simulink model "System_Analysis_for_no_P_and_PI_Controllers"  (R2023a)
settings: Solver=FixedStepDiscrete  StartTime=0.0  StopTime=100  FixedStep=0.001  RelTol=1e-3  EnableMultiTasking=on
undefined symbols (not defined in the file or in its folder): DiscIntNeverNeededParam
libraries: arduinolib x6
settings Model: ExtModeTrigDuration=2  Creator=Mohamed Ezzelrgal  LastModifiedBy=Mohamed Ezzelrgal
settings OptimizationCC: EnhancedBackFolding=on  PassReuseOutputArgsAs=Individual arguments  ZeroExternalMemoryAtStartup=off  ZeroInternalMemoryAtStartup=off  MaxStackSize=64  OptimizeBlockOrder=speed  DifferentSizesBufferReuse=on  OptimizationCustomize=off  EfficientTunableParamExpr=on
settings DebuggingCC: ParameterTunabilityLossMsg=error
settings HardwareCC: ProdBitPerInt=16  ProdBitPerPointer=16  ProdBitPerSizeT=16  ProdBitPerPtrDiffT=16  ProdLargestAtomicFloat=None  ProdWordSize=8  ProdHWDeviceType=Atmel->AVR
settings SFSimCC: MATLABDynamicMemAlloc=off
settings RTWCC: Description=Embedded Coder  SystemTargetFile=ert.tlc  HardwareBoard=Arduino Uno  TemplateMakefile=ert_default_tmf  Toolchain=Arduino AVR  BuildConfiguration=Faster Runs
settings CodeAppCC: ForceParamTrailComments=on  IgnoreCustomStorageClasses=off  OperatorAnnotations=on  SimulinkDataObjDesc=on  SFDataObjDesc=on  InsertBlockDesc=on
settings ERTTargetCC: SupportContinuousTime=on  SupportVariableSizeSignals=on  ExtModeTransport=3  ExtModeStaticAlloc=on  ExtModeAutomaticAllocSize=off  ExtModeStaticAllocSize=250  ExtModeMexFile=ext_xcp  ExtModeIntrfLevel=Level2 - Open

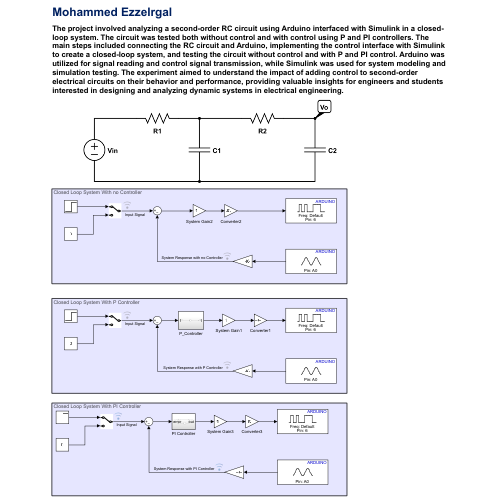
[thumbnail: Simulink's stored preview of the top-level diagram]
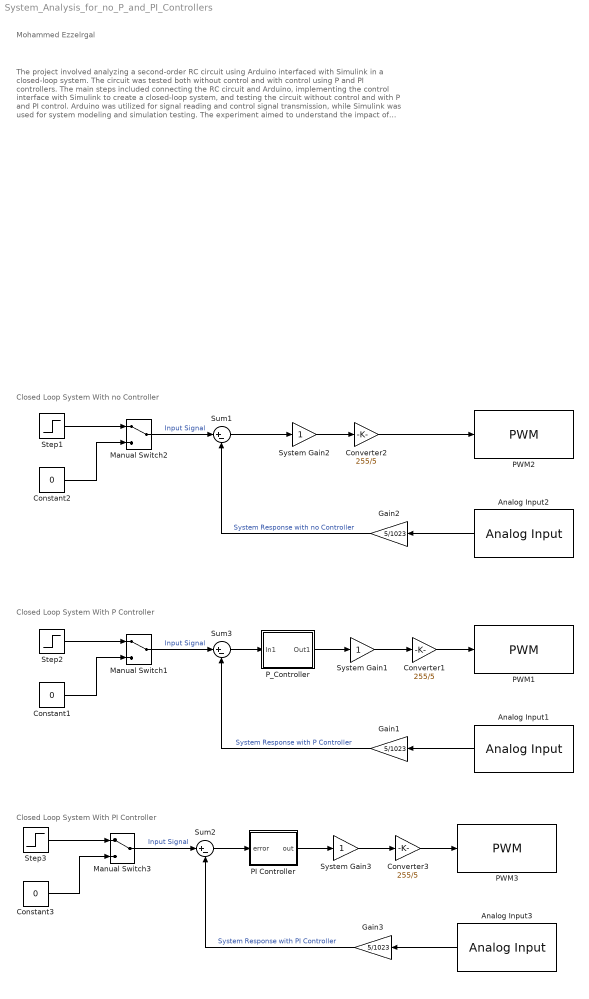
== system System_Analysis_for_no_P_and_PI_Controllers ==
  note: The project involved analyzing a second-order RC circuit using Arduino interfaced with Simulink in a closed-loop system. The circuit was tested both without control and with control using P and PI controllers. The main steps included connecting the RC circuit and Arduino, implementing the control interface with Simulink to create a closed-loop system, and testing the circuit without control and with P and PI control. Arduino was utilized for signal reading and control signal transmission, while Simulink was used for system modeling and simulation testing. The experiment aimed to understand the impact of adding control to second-order electrical circuits on their behavior and performance, providing valuable insights for engineers and students interested in designing and analyzing dynamic systems in electrical engineering.
  note: Mohammed Ezzelrgal
  note: Closed Loop System With PI Controller
  note: Closed Loop System With P Controller
  note: Closed Loop System With no Controller
  Analog Input1 : arduinolib/Analog Input  pinNumber=0  ReadResultsOnly=off  ConversionTriggerSource=Software  ExternalTriggerType=uint32( 0 )  OutputDataType=uint16  EnableConversionCompleteNotify=off  EnableOuputStatus=off  SampleTime=-1  blockPlatform=arduino
  Analog Input2 : arduinolib/Analog Input  pinNumber=0  ReadResultsOnly=off  ConversionTriggerSource=Software  ExternalTriggerType=uint32( 0 )  OutputDataType=uint16  EnableConversionCompleteNotify=off  EnableOuputStatus=off  SampleTime=-1  blockPlatform=arduino
  Analog Input3 : arduinolib/Analog Input  pinNumber=0  ReadResultsOnly=off  ConversionTriggerSource=Software  ExternalTriggerType=uint32( 0 )  OutputDataType=uint16  EnableConversionCompleteNotify=off  EnableOuputStatus=off  SampleTime=-1  blockPlatform=arduino
  Constant1 : Constant  Value=0
  Constant2 : Constant  Value=0
  Constant3 : Constant  Value=0
  Converter1 : Gain  Gain=255/5
  Converter2 : Gain  Gain=255/5
  Converter3 : Gain  Gain=255/5
  Gain1 : Gain  Gain=5/1023
  Gain2 : Gain  Gain=5/1023
  Gain3 : Gain  Gain=5/1023
  Manual Switch1 : ManualSwitch
  Manual Switch2 : ManualSwitch
  Manual Switch3 : ManualSwitch
  PI Controller : Subsystem
  PWM1 : arduinolib/PWM  pinNumber=6  frequencyType=Default  desiredFrequency=490.2  achievableFrequency=490.2
  PWM2 : arduinolib/PWM  pinNumber=6  frequencyType=Default  desiredFrequency=490.2  achievableFrequency=490.2
  PWM3 : arduinolib/PWM  pinNumber=6  frequencyType=Default  desiredFrequency=490.2  achievableFrequency=490.2
  P_Controller : Subsystem
  Step1 : Step  SampleTime=0
  Step2 : Step  SampleTime=0
  Step3 : Step  SampleTime=0
  Sum1 : Sum  Inputs=|+-
  Sum2 : Sum  Inputs=|+-
  Sum3 : Sum  Inputs=|+-
  System Gain1 : Gain
  System Gain2 : Gain
  System Gain3 : Gain
  wires:
  Analog Input1/1 -> Gain1/1
  Manual Switch1/1 -> Sum3/1  "Input Signal"
  Converter1/1 -> PWM1/1
  Sum3/1 -> P_Controller/1(In1)
  Step2/1 -> Manual Switch1/1
  Constant1/1 -> Manual Switch1/2
  P_Controller/1(Out1) -> System Gain1/1
  System Gain1/1 -> Converter1/1
  Gain1/1 -> Sum3/2  "System Response with P Controller"
  Gain2/1 -> Sum1/2  "System Response with no Controller"
  System Gain2/1 -> Converter2/1
  Constant2/1 -> Manual Switch2/2
  Step1/1 -> Manual Switch2/1
  Converter2/1 -> PWM2/1
  Manual Switch2/1 -> Sum1/1  "Input Signal"
  Analog Input2/1 -> Gain2/1
  Sum1/1 -> System Gain2/1
  Constant3/1 -> Manual Switch3/2
  Step3/1 -> Manual Switch3/1
  Sum2/1 -> PI Controller/1(error)
  Manual Switch3/1 -> Sum2/1  "Input Signal"
  Gain3/1 -> Sum2/2  "System Response with PI Controller"
  System Gain3/1 -> Converter3/1
  PI Controller/1(out) -> System Gain3/1
  Converter3/1 -> PWM3/1
  Analog Input3/1 -> Gain3/1

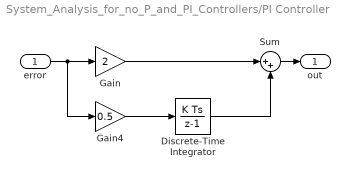
== system System_Analysis_for_no_P_and_PI_Controllers/PI Controller ==
  error : Inport
  Discrete-Time Integrator : DiscreteIntegrator  SampleTime=-1  ICPrevOutput=DiscIntNeverNeededParam  ICPrevScaledInput=DiscIntNeverNeededParam
  Gain : Gain  Gain=2
  Gain4 : Gain  Gain=0.5
  Sum : Sum  Inputs=|++
  out : Outport
  wires:
  error/1 -> Gain4/1, Gain/1
  Gain/1 -> Sum/1
  Gain4/1 -> Discrete-Time Integrator/1
  Discrete-Time Integrator/1 -> Sum/2
  Sum/1 -> out/1

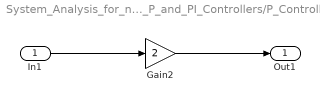
== system System_Analysis_for_no_P_and_PI_Controllers/P_Controller ==
  In1 : Inport
  Gain2 : Gain  Gain=2
  Out1 : Outport
  wires:
  In1/1 -> Gain2/1
  Gain2/1 -> Out1/1
